simulink model "acionamento_vetorial1"  (Simulink 8.0)
settings: Solver=ode45  StartTime=0.0  StopTime=5  MaxStep=1e-4  RelTol=1e-3
libraries: BLDC x3
settings Model: Creator=Rodrigo  LastModifiedBy=h3now
settings DataIOCC: SignalLoggingSaveFormat=ModelDataLogs
settings DebuggingCC: FcnCallInpInsideContextMsg=EnableAllAsWarning
settings GRTTargetCC: CombineOutputUpdateFcns=off  GRTInterface=on
settings ConfigurationSet: Description=SimMechanics 2G

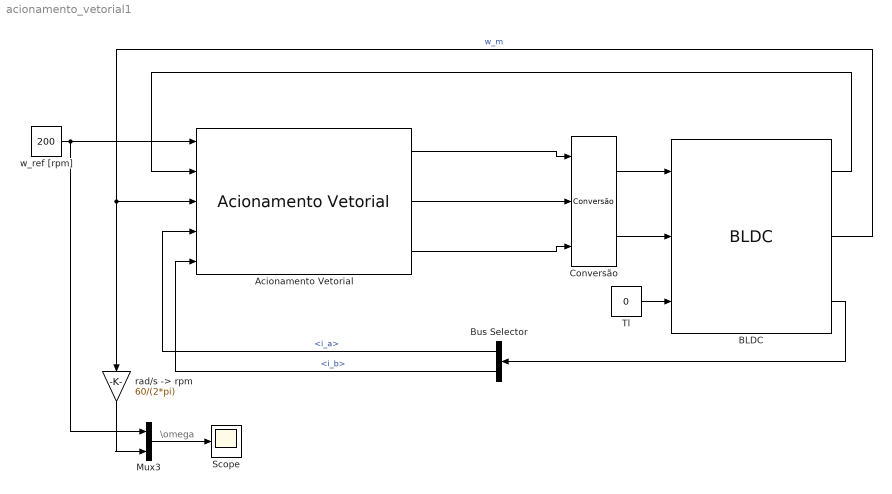
== system acionamento_vetorial1 ==
  note: \omega
  Acionamento Vetorial : BLDC/Acionamento Vetorial  P=8
  BLDC : BLDC/BLDC  J=3.84e-7 + 1e-4  R=23.9/2  L=2.35e-3/2  P=8  Kt=11.3e-3  Ke=11.3e-3  Kd=0  F_stick=0  F_slip=0  default_fcem=on  fcem_a=fcem_a  fcem_b=fcem_b  fcem_c=fcem_c
  Bus Selector : BusSelector  OutputSignals=Correntes.i_a,Correntes.i_b
  Conversão : BLDC/Conversão
  Mux3 : Mux  Inputs=2
  Scope : Scope
      settings: TimeRange=10  YMin=20  YMax=200  Decimation=10
  Tl : Constant  Value=0
  "rad/s -> rpm" : Gain  Gain=60/(2*pi)
  w_ref [rpm] : Constant  Value=200
  wires:
  BLDC/3 -> Bus Selector/1
  Tl/1 -> BLDC/3
  Mux3/1 -> Scope/1
  BLDC/1 -> Acionamento Vetorial/2
  BLDC/2 -> Acionamento Vetorial/3, "rad/s -> rpm"/1  "w_m"
  w_ref [rpm]/1 -> Acionamento Vetorial/1, Mux3/1
  "rad/s -> rpm"/1 -> Mux3/2
  Bus Selector/1 -> Acionamento Vetorial/4  "<i_a>"
  Bus Selector/2 -> Acionamento Vetorial/5  "<i_b>"
  Conversão/1 -> BLDC/1
  Conversão/2 -> BLDC/2
  Acionamento Vetorial/1 -> Conversão/1
  Acionamento Vetorial/2 -> Conversão/2
  Acionamento Vetorial/3 -> Conversão/3
